simulink model "cv_1_sim"  (R2019b)
settings: Solver=FixedStepAuto  StartTime=0.0  StopTime=Tsim  FixedStep=Ts  RelTol=1e-3
values from neighbouring files (symbols this model uses):
  C = C_vec(i)    [cv_1.m]
  R = R_vec(i)    [cv_1.m]
  u_0 = u_0_vec(i)    [cv_1.m]
settings Model: Creator=Martin Dodek  LastModifiedBy=Martin Dodek

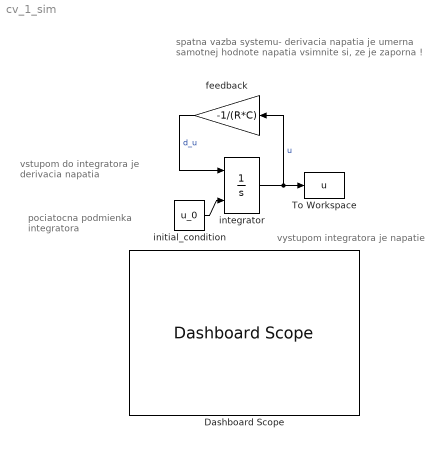
== system cv_1_sim ==
  note: vystupom integratora je napatie
  note: spatna vazba systemu-
      | derivacia napatia je umerna samotnej hodnote napatia
      | vsimnite si, ze je zaporna !
  note: vstupom do integratora
      | je derivacia napatia
  note: pociatocna
      | podmienka integratora
  Dashboard Scope : DashboardScope
  To Workspace : ToWorkspace  VariableName=u  SampleTime=-1
  feedback : Gain  Gain=-1/(R*C)
  initial_condition : Constant  Value=u_0
  integrator : Integrator  InitialConditionSource=external  InitialCondition=u_0
  wires:
  initial_condition/1 -> integrator/2
  integrator/1 -> To Workspace/1, feedback/1  "u"
  feedback/1 -> integrator/1  "d_u"
